simulink model "ph_I_ph"  (R2017b)
settings: Solver=VariableStepAuto  StartTime=0.0  StopTime=10.0  RelTol=1e-3
settings Model: Creator=yaakovazat  LastModifiedBy=yaakovazat

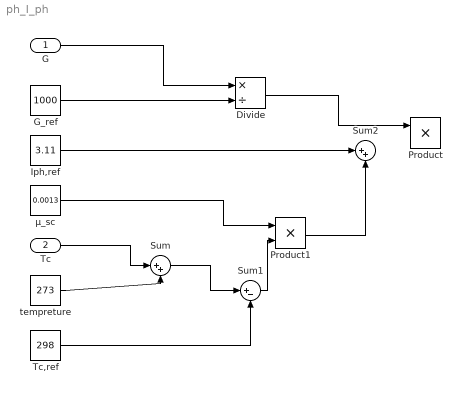
== system ph_I_ph ==
  G : Inport
  Tc : Inport  Port=2
  Divide : Product  Inputs=*/
  G_ref : Constant  Value=1000
  Iph,ref : Constant  Value=3.11
  Product : Product
  Product1 : Product
  Sum : Sum  Inputs=|++
  Sum1 : Sum  Inputs=|+-
  Sum2 : Sum  Inputs=|++
  Tc,ref : Constant  Value=298
  tempreture : Constant  Value=273
  μ_sc : Constant  Value=0.0013
  wires:
  G_ref/1 -> Divide/2
  G/1 -> Divide/1
  Divide/1 -> Product/1
  Tc/1 -> Sum/1
  tempreture/1 -> Sum/2
  Tc,ref/1 -> Sum1/2
  Sum/1 -> Sum1/1
  μ_sc/1 -> Product1/1
  Sum1/1 -> Product1/2
  Product1/1 -> Sum2/2
  Iph,ref/1 -> Sum2/1
